simulink model "simulator1"  (R2023b)
settings: Solver=VariableStepAuto  StartTime=0.0  StopTime=10  MaxStep=1e-5  RelTol=1e-3
undefined symbols (not defined in the file): ke, p
libraries: simulink x2
settings Model: Creator=miqui  LastModifiedBy=miqui

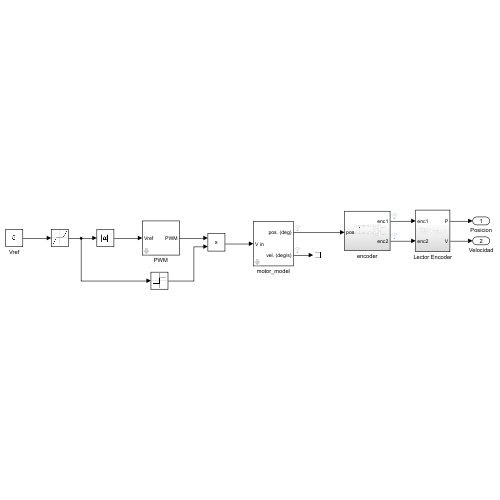
[thumbnail: Simulink's stored preview of the top-level diagram]
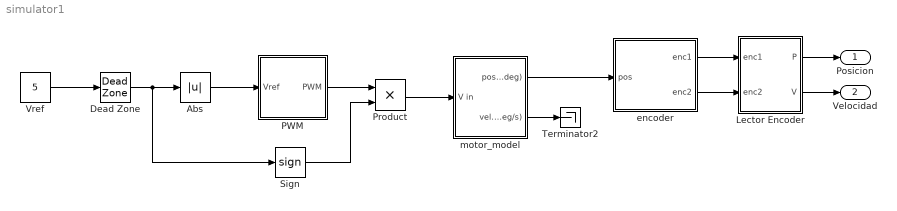
== system simulator1 ==
  Abs : Abs  SaturateOnIntegerOverflow=off
  Dead Zone : DeadZone
  Lector Encoder : Subsystem
  PWM : Subsystem  mask{T=1e-3, Vmax=12}
      mask prompts: T "Periodo"; Vmax "Voltaje máximo"
  Product : Product
  Sign : Signum
  Terminator2 : Terminator
  Vref : Constant  Value=5
  encoder : Subsystem
  motor_model : Subsystem  mask{k_e=ke, p=p}
  Posicion : Outport
  Velocidad : Outport  Port=2
  wires:
  Dead Zone/1 -> Sign/1, Abs/1
  Abs/1 -> PWM/1(Vref)
  PWM/1(PWM) -> Product/1
  Product/1 -> motor_model/1(V in)
  Sign/1 -> Product/2
  Vref/1 -> Dead Zone/1
  encoder/1(enc1) -> Lector Encoder/1(enc1)
  encoder/2(enc2) -> Lector Encoder/2(enc2)
  Lector Encoder/2(V) -> Velocidad/1
  Lector Encoder/1(P) -> Posicion/1
  motor_model/2(vel. (deg/s)) -> Terminator2/1
  motor_model/1(pos. (deg)) -> encoder/1(pos)

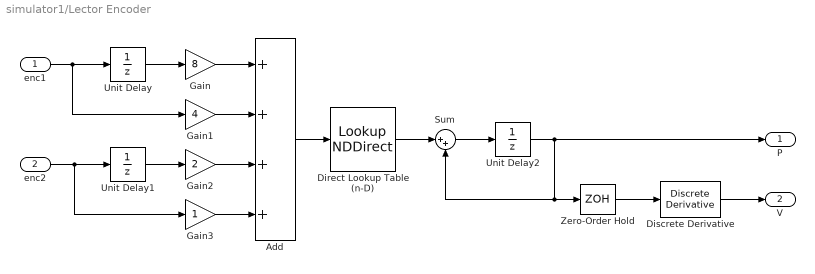
== system simulator1/Lector Encoder ==
  enc1 : Inport
  enc2 : Inport  Port=2
  Add : Sum  Inputs=++++  OutDataTypeStr=double
  Direct Lookup Table (n-D) : LookupNDDirect  NumberOfTableDimensions=1  Table=[0,-1,1,0,1,0,0,-1,-1,0,0,1,0,1,-1,0]
  Discrete Derivative : simulink/Discrete/Discrete Derivative  gainval=1.0  ICPrevScaledInput=0.0  OutMin=[]  OutMax=[]  OutDataType=fixdt(1, 16)  OutScaling=2^-10  DoSatur=off
  Gain : Gain  Gain=8
  Gain1 : Gain  Gain=4
  Gain2 : Gain  Gain=2
  Gain3 : Gain
  Sum : Sum  Inputs=|++
  Unit Delay : UnitDelay  SampleTime=-1  HasFrameUpgradeWarning=on
  Unit Delay1 : UnitDelay  SampleTime=-1  HasFrameUpgradeWarning=on
  Unit Delay2 : UnitDelay  SampleTime=-1  HasFrameUpgradeWarning=on
  Zero-Order Hold : ZeroOrderHold  SampleTime=0.01
  P : Outport
  V : Outport  Port=2
  wires:
  enc1/1 -> Gain1/1, Unit Delay/1
  enc2/1 -> Gain3/1, Unit Delay1/1
  Unit Delay/1 -> Gain/1
  Unit Delay1/1 -> Gain2/1
  Gain/1 -> Add/1
  Gain1/1 -> Add/2
  Gain2/1 -> Add/3
  Gain3/1 -> Add/4
  Add/1 -> Direct Lookup Table (n-D)/1
  Direct Lookup Table (n-D)/1 -> Sum/1
  Sum/1 -> Unit Delay2/1
  Unit Delay2/1 -> Zero-Order Hold/1, Sum/2, P/1
  Zero-Order Hold/1 -> Discrete Derivative/1
  Discrete Derivative/1 -> V/1

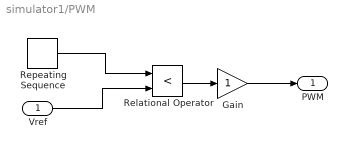
== system simulator1/PWM ==
  Vref : Inport
  Gain : Gain
  Relational Operator : RelationalOperator  Operator=<  OutDataTypeStr=boolean  RndMeth=Simplest  InputSameDT=off
  Repeating Sequence : simulink/Sources/Repeating Sequence  rep_seq_t=linspace(0,T,100)  rep_seq_y=linspace(0,Vmax,100)
  PWM : Outport
  wires:
  Relational Operator/1 -> Gain/1
  Gain/1 -> PWM/1
  Vref/1 -> Relational Operator/2
  Repeating Sequence/1 -> Relational Operator/1

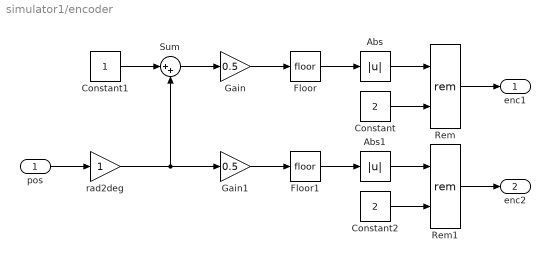
== system simulator1/encoder ==
  pos : Inport
  Abs : Abs  SaturateOnIntegerOverflow=off
  Abs1 : Abs  SaturateOnIntegerOverflow=off
  Constant : Constant  Value=2
  Constant1 : Constant
  Constant2 : Constant  Value=2
  Floor : Rounding
  Floor1 : Rounding
  Gain : Gain  Gain=0.5
  Gain1 : Gain  Gain=0.5
  Rem : Math  Operator=rem
  Rem1 : Math  Operator=rem
  Sum : Sum  Inputs=|++
  rad2deg : Gain
  enc1 : Outport
  enc2 : Outport  Port=2
  wires:
  pos/1 -> rad2deg/1
  Rem/1 -> enc1/1
  Abs/1 -> Rem/1
  Constant/1 -> Rem/2
  Floor/1 -> Abs/1
  Gain/1 -> Floor/1
  Sum/1 -> Gain/1
  Constant1/1 -> Sum/1
  Gain1/1 -> Floor1/1
  Constant2/1 -> Rem1/2
  Floor1/1 -> Abs1/1
  Rem1/1 -> enc2/1
  Abs1/1 -> Rem1/1
  rad2deg/1 -> Sum/2, Gain1/1

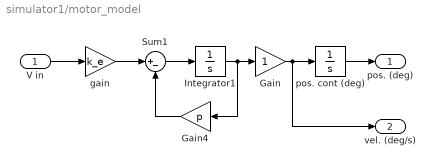
== system simulator1/motor_model ==
  V in : Inport
  Gain : Gain
  Gain4 : Gain  Gain=p
  Integrator1 : Integrator
  Sum1 : Sum  Inputs=|+-
  gain : Gain  Gain=k_e
  pos. cont (deg) : Integrator
  pos. (deg) : Outport
  vel. (deg/s) : Outport  Port=2
  wires:
  Sum1/1 -> Integrator1/1
  Gain4/1 -> Sum1/2
  Integrator1/1 -> Gain/1, Gain4/1
  gain/1 -> Sum1/1
  V in/1 -> gain/1
  Gain/1 -> pos. cont (deg)/1, vel. (deg/s)/1
  pos. cont (deg)/1 -> pos. (deg)/1
